simulink model "CM340A_AdcDiagc"
settings: Solver=FixedStepDiscrete  SolverMode=SingleTasking  StartTime=0.0  StopTime=1  FixedStep=0.002  RelTol=1e-3
values from neighbouring files (symbols this model uses):
  Adc0Diagc = DataDict.NTC    [CM340A_AdcDiagc_DataDict.m]
  Adc1Diagc = DataDict.NTC    [CM340A_AdcDiagc_DataDict.m]
  ADCDIAG0REFVOLT_VOLT_F32 = DataDict.Constant    [CM340A_AdcDiagc_DataDict.m]
  ADCDIAG2REFVOLT_VOLT_F32 = DataDict.Constant    [CM340A_AdcDiagc_DataDict.m]
  ADCDIAG4REFVOLT_VOLT_F32 = DataDict.Constant    [CM340A_AdcDiagc_DataDict.m]
  AdcDiagcNtc0x032FailStep = DataDict.Calibration    [CM340A_AdcDiagc_DataDict.m]
  AdcDiagcNtc0x032PassStep = DataDict.Calibration    [CM340A_AdcDiagc_DataDict.m]
  AdcDiagcNtc0x033FailStep = DataDict.Calibration    [CM340A_AdcDiagc_DataDict.m]
  AdcDiagcNtc0x033PassStep = DataDict.Calibration    [CM340A_AdcDiagc_DataDict.m]
  AdcDiagcSt = DataDict.PIM    [CM340A_AdcDiagc_DataDict.m]
  ADCDIAGPARFLTPRM_CNT_U08 = DataDict.Constant    [CM340A_AdcDiagc_DataDict.m]
  ADCDIAGSCANGROUP2REFFLTPRM_CNT_U08 = DataDict.Constant    [CM340A_AdcDiagc_DataDict.m]
  ADCDIAGSCANGROUP3REFFLTPRM_CNT_U08 = DataDict.Constant    [CM340A_AdcDiagc_DataDict.m]
  ADCDIAGSCANGROUPENDREFVOLT_VOLT_F32 = DataDict.Constant    [CM340A_AdcDiagc_DataDict.m]
  ADCDIAGSCANGROUPSTRTREFVOLT_VOLT_F32 = DataDict.Constant    [CM340A_AdcDiagc_DataDict.m]
  ADCDNECRPARERRCLR_CNT_U08 = DataDict.Constant    [CM340A_AdcDiagc_DataDict.m]
  ADCDNPERPARERRMASK_CNT_U08 = DataDict.Constant    [CM340A_AdcDiagc_DataDict.m]
  VIRTCH21_CNT_U08 = DataDict.Constant    [CM340A_AdcDiagc_DataDict.m]
  VIRTCH22_CNT_U08 = DataDict.Constant    [CM340A_AdcDiagc_DataDict.m]
  VIRTCH23_CNT_U08 = DataDict.Constant    [CM340A_AdcDiagc_DataDict.m]
undefined symbols (not defined in the file or in its folder): NtcSts1, sigbuilder_block, SigQlfr1
libraries: simulink x42, CM340A_AdcDiagc_Library x40
(part 3 of 4)

== system CM340A_AdcDiagc/AdcDiagc/AdcDiagcPer1/Adc Daigc Pointer/Strt & End Ptr Store/State 4 ==
  Action Port : ActionPort  ActionType=elseif
  Constant3 : Constant  Value=VIRTCH22_CNT_U08
  Constant4 : Constant  Value=VIRTCH22_CNT_U08
  CopyRight2 : Subsystem  Description=|  mask(Copyright Information){none=on}
      | Copyright info block.                                               
      |                                                                     
      | Place copyright information at the top of every subsystem in design.
      mask prompts: none "No parameters"
      mask help: Place copyright information at the top of every subsystem in design.
      mask Display:
      | NxtrConf = 'Nexteer Confidential';
      | 
      | sys = bdroot; %handle for the current model ("system")
      | first = get_param(sys,'Created');
      | first = first(end-3:end);  %year is last four digits
      | 
      | last = get_param(sys,'LastModifiedDate');
      | if isempty(last)
      |     last = datestr(now,'yyyy');
      | else
      |     last = last(end-3:end);
      | end
      | 
      | if strcmp(first,last)
      |     fprintf('%s -- Copyright %s Nexteer',NxtrConf,first)
      | else
      |     fprintf('%s -- %s%s- %s Nexteer',NxtrConf,char(169),first,last)
      | end
  AdcDiagcStrtPtr : Outport
  AdcDiagcEndPtr : Outport  Port=2
  wires:
  Constant3/1 -> AdcDiagcStrtPtr/1
  Constant4/1 -> AdcDiagcEndPtr/1

== system CM340A_AdcDiagc/AdcDiagc/AdcDiagcPer1/Adc Daigc Pointer/Strt & End Ptr Store/State 6 ==
  Action Port : ActionPort  ActionType=elseif
  Constant3 : Constant  Value=VIRTCH21_CNT_U08
  Constant4 : Constant  Value=VIRTCH23_CNT_U08
  CopyRight2 : Subsystem  Description=|  mask(Copyright Information){none=on}
      | Copyright info block.                                               
      |                                                                     
      | Place copyright information at the top of every subsystem in design.
      mask prompts: none "No parameters"
      mask help: Place copyright information at the top of every subsystem in design.
      mask Display:
      | NxtrConf = 'Nexteer Confidential';
      | 
      | sys = bdroot; %handle for the current model ("system")
      | first = get_param(sys,'Created');
      | first = first(end-3:end);  %year is last four digits
      | 
      | last = get_param(sys,'LastModifiedDate');
      | if isempty(last)
      |     last = datestr(now,'yyyy');
      | else
      |     last = last(end-3:end);
      | end
      | 
      | if strcmp(first,last)
      |     fprintf('%s -- Copyright %s Nexteer',NxtrConf,first)
      | else
      |     fprintf('%s -- %s%s- %s Nexteer',NxtrConf,char(169),first,last)
      | end
  AdcDiagcStrtPtr : Outport
  AdcDiagcEndPtr : Outport  Port=2
  wires:
  Constant3/1 -> AdcDiagcStrtPtr/1
  Constant4/1 -> AdcDiagcEndPtr/1

== system CM340A_AdcDiagc/AdcDiagc/AdcDiagcPer1/Adc0 Diagc/Adc0 Scan Group Strt and End Ref Voltage Diagc/CopyRight2 ==

== system CM340A_AdcDiagc/AdcDiagc/AdcDiagcPer1/Adc0 Diagc/Adc0 Scan Group Strt and End Ref Voltage Diagc/Subsystem ==
  Parameter Byte : Inport
  FltCntrPrev : Inport  Port=2
  Add : Sum
  Bitwise Operator : simulink/Logic and Bit Operations/Bitwise Operator  logicop=AND  UseBitMask=off  NumInputPorts=2  BitMask=bin2dec('01111111')  BitMaskRealWorld=Stored Integer
  Constant : Constant  Value=0
  Constant1 : Constant  Value=127  OutDataTypeStr=uint8
  CopyRight2 : Subsystem  Description=|  mask(Copyright Information){none=on}
      | Copyright info block.                                               
      |                                                                     
      | Place copyright information at the top of every subsystem in design.
      mask prompts: none "No parameters"
      mask help: Place copyright information at the top of every subsystem in design.
      mask Display:
      | NxtrConf = 'Nexteer Confidential';
      | 
      | sys = bdroot; %handle for the current model ("system")
      | first = get_param(sys,'Created');
      | first = first(end-3:end);  %year is last four digits
      | 
      | last = get_param(sys,'LastModifiedDate');
      | if isempty(last)
      |     last = datestr(now,'yyyy');
      | else
      |     last = last(end-3:end);
      | end
      | 
      | if strcmp(first,last)
      |     fprintf('%s -- Copyright %s Nexteer',NxtrConf,first)
      | else
      |     fprintf('%s -- %s%s- %s Nexteer',NxtrConf,char(169),first,last)
      | end
  Data Type Conversion2 : DataTypeConversion  OutDataTypeStr=uint8
  Relational Operator : RelationalOperator  Operator=>  OutDataTypeStr=boolean
  Scope1 : Scope  NumInputPorts=2
      settings: ShowLegends=on  TimeRange=1000  YMin=-2~0  YMax=2~256  SaveName=ScopeData3
  FltCntr : Outport
  wires:
  Constant/1 -> Relational Operator/2
  Parameter Byte/1 -> Scope1/1, Relational Operator/1
  Relational Operator/1 -> Data Type Conversion2/1
  Add/1 -> Bitwise Operator/1
  Bitwise Operator/1 -> FltCntr/1, Scope1/2
  FltCntrPrev/1 -> Add/2
  Data Type Conversion2/1 -> Add/1
  Constant1/1 -> Bitwise Operator/2

== system CM340A_AdcDiagc/AdcDiagc/AdcDiagcPer1/Adc0 Diagc/Adc0 Scan Group Strt and End Ref Voltage Diagc/Subsystem1 ==
  Parameter Byte : Inport
  FltCntrPrev : Inport  Port=2
  Add : Sum
  Bitwise Operator : simulink/Logic and Bit Operations/Bitwise Operator  logicop=AND  UseBitMask=off  NumInputPorts=2  BitMask=bin2dec('01111111')  BitMaskRealWorld=Stored Integer
  Constant : Constant  Value=0
  Constant1 : Constant  Value=127  OutDataTypeStr=uint8
  CopyRight2 : Subsystem  Description=|  mask(Copyright Information){none=on}
      | Copyright info block.                                               
      |                                                                     
      | Place copyright information at the top of every subsystem in design.
      mask prompts: none "No parameters"
      mask help: Place copyright information at the top of every subsystem in design.
      mask Display:
      | NxtrConf = 'Nexteer Confidential';
      | 
      | sys = bdroot; %handle for the current model ("system")
      | first = get_param(sys,'Created');
      | first = first(end-3:end);  %year is last four digits
      | 
      | last = get_param(sys,'LastModifiedDate');
      | if isempty(last)
      |     last = datestr(now,'yyyy');
      | else
      |     last = last(end-3:end);
      | end
      | 
      | if strcmp(first,last)
      |     fprintf('%s -- Copyright %s Nexteer',NxtrConf,first)
      | else
      |     fprintf('%s -- %s%s- %s Nexteer',NxtrConf,char(169),first,last)
      | end
  Data Type Conversion2 : DataTypeConversion  OutDataTypeStr=uint8
  Relational Operator : RelationalOperator  Operator=>  OutDataTypeStr=boolean
  Scope1 : Scope  NumInputPorts=2
      settings: ShowLegends=on  TimeRange=1000  YMin=-2~0  YMax=2~256  SaveName=ScopeData4
  FltCntr : Outport
  wires:
  Constant/1 -> Relational Operator/2
  Parameter Byte/1 -> Scope1/1, Relational Operator/1
  Relational Operator/1 -> Data Type Conversion2/1
  Add/1 -> Bitwise Operator/1
  Bitwise Operator/1 -> FltCntr/1, Scope1/2
  FltCntrPrev/1 -> Add/2
  Data Type Conversion2/1 -> Add/1
  Constant1/1 -> Bitwise Operator/2

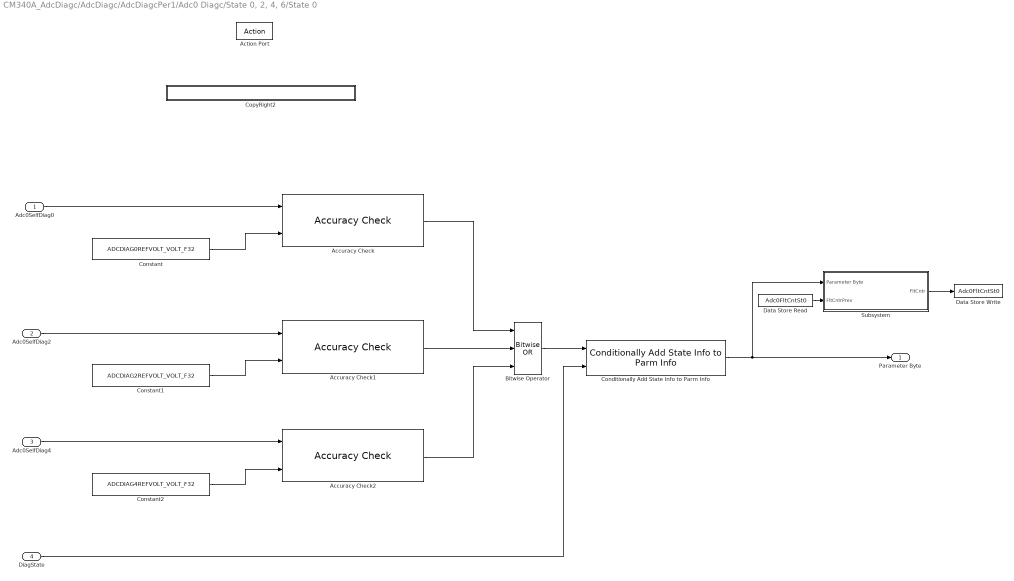
== system CM340A_AdcDiagc/AdcDiagc/AdcDiagcPer1/Adc0 Diagc/State 0, 2, 4, 6/State 0 ==
  Adc0SelfDiag0 : Inport  RequirementInfo={} %GIDa_a23626af_39b5_4ed6_8e27_9b4935a63c0c
  Adc0SelfDiag2 : Inport  RequirementInfo={} %GIDa_c5f8a541_29c5_4f9c_88e4_ee09e309bb5e  Port=2
  Adc0SelfDiag4 : Inport  RequirementInfo={} %GIDa_cb51580b_1e3d_432c_bc7e_60394d016f61  Port=3
  DiagState : Inport  Port=4
  Action Port : ActionPort  ActionType=then
  Accuracy Check : CM340A_AdcDiagc_Library/Accuracy Check  RequirementInfo="{'linktype_rmi_doors' '000079f2 (/ESG Group/FDD Module Requirements/EA4 Specific/CM340A_AdcDiagc)' '#CM340A_190' 'true' 'REQ:  CM340A_190' '' } %GIDa_1e4f0f1f_efcc_4971_978e_b5150d55866c"
  Accuracy Check1 : CM340A_AdcDiagc_Library/Accuracy Check  RequirementInfo="{'linktype_rmi_doors' '000079f2 (/ESG Group/FDD Module Requirements/EA4 Specific/CM340A_AdcDiagc)' '#CM340A_191' 'true' 'REQ:  CM340A_191' '' } %GIDa_c4102599_b47c_4dea_9090_c33325f35ddf"
  Accuracy Check2 : CM340A_AdcDiagc_Library/Accuracy Check  RequirementInfo="{'linktype_rmi_doors' '000079f2 (/ESG Group/FDD Module Requirements/EA4 Specific/CM340A_AdcDiagc)' '#CM340A_192' 'true' 'REQ:  CM340A_192' '' } %GIDa_02166258_10fd_4a19_8760_8d3e602927dd"
  Bitwise Operator : simulink/Logic and Bit Operations/Bitwise Operator  logicop=OR  UseBitMask=off  NumInputPorts=3  BitMask=bin2dec('11011001')  BitMaskRealWorld=Stored Integer
  Conditionally Add State Info to Parm Info : CM340A_AdcDiagc_Library/Conditionally Add State Info to Parm Info  RequirementInfo="{'linktype_rmi_doors' '000079f2 (/ESG Group/FDD Module Requirements/EA4 Specific/CM340A_AdcDiagc)' '#CM340A_173' 'true' 'REQ:  CM340A_173' '' } %GIDa_80ab0b66_9e6f_4bf7_ac53_ccce88f803b6"
  Constant : Constant  Value=ADCDIAG0REFVOLT_VOLT_F32
  Constant1 : Constant  Value=ADCDIAG2REFVOLT_VOLT_F32
  Constant2 : Constant  Value=ADCDIAG4REFVOLT_VOLT_F32
  CopyRight2 : Subsystem  Description=|  mask(Copyright Information){none=on}
      | Copyright info block.                                               
      |                                                                     
      | Place copyright information at the top of every subsystem in design.
      mask prompts: none "No parameters"
      mask help: Place copyright information at the top of every subsystem in design.
      mask Display:
      | NxtrConf = 'Nexteer Confidential';
      | 
      | sys = bdroot; %handle for the current model ("system")
      | first = get_param(sys,'Created');
      | first = first(end-3:end);  %year is last four digits
      | 
      | last = get_param(sys,'LastModifiedDate');
      | if isempty(last)
      |     last = datestr(now,'yyyy');
      | else
      |     last = last(end-3:end);
      | end
      | 
      | if strcmp(first,last)
      |     fprintf('%s -- Copyright %s Nexteer',NxtrConf,first)
      | else
      |     fprintf('%s -- %s%s- %s Nexteer',NxtrConf,char(169),first,last)
      | end
  Data Store Read : DataStoreRead  DataStoreName=Adc0FltCntSt0
  Data Store Write : DataStoreWrite  DataStoreName=Adc0FltCntSt0
  Subsystem : Subsystem
  Parameter Byte : Outport
  wires:
  Adc0SelfDiag0/1 -> Accuracy Check/1
  Constant/1 -> Accuracy Check/2
  Adc0SelfDiag2/1 -> Accuracy Check1/1
  Constant1/1 -> Accuracy Check1/2
  Adc0SelfDiag4/1 -> Accuracy Check2/1
  Constant2/1 -> Accuracy Check2/2
  Accuracy Check/1 -> Bitwise Operator/1
  Accuracy Check1/1 -> Bitwise Operator/2
  Accuracy Check2/1 -> Bitwise Operator/3
  Conditionally Add State Info to Parm Info/1 -> Subsystem/1(Parameter Byte), Parameter Byte/1
  Subsystem/1(FltCntr) -> Data Store Write/1
  Data Store Read/1 -> Subsystem/2(FltCntrPrev)
  DiagState/1 -> Conditionally Add State Info to Parm Info/2
  Bitwise Operator/1 -> Conditionally Add State Info to Parm Info/1

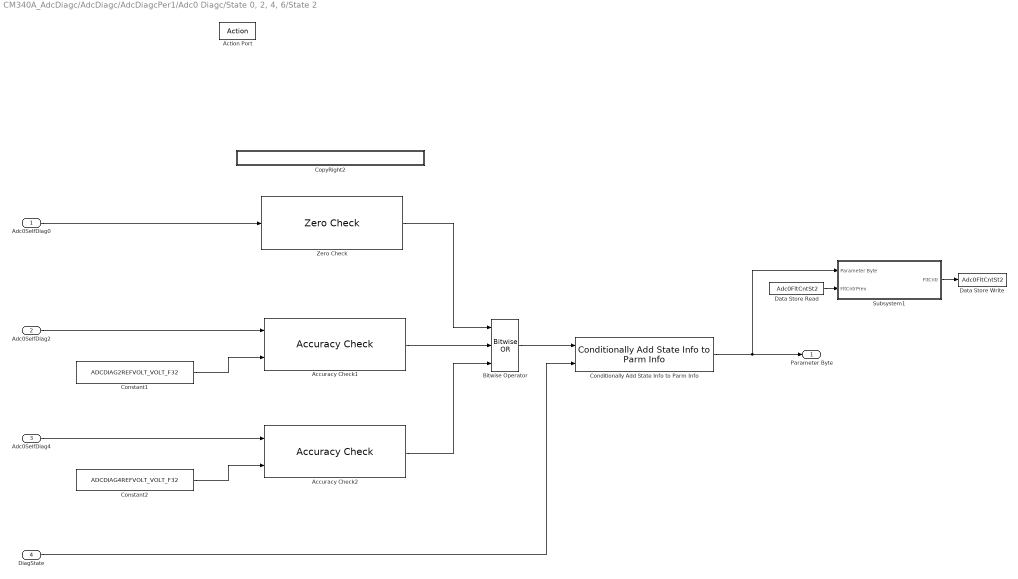
== system CM340A_AdcDiagc/AdcDiagc/AdcDiagcPer1/Adc0 Diagc/State 0, 2, 4, 6/State 2 ==
  Adc0SelfDiag0 : Inport  RequirementInfo={} %GIDa_e1135336_cc92_42c6_b177_9493a56e2976
  Adc0SelfDiag2 : Inport  RequirementInfo={} %GIDa_5cb7465b_8501_4efa_b631_17bf9f2d25f9  Port=2
  Adc0SelfDiag4 : Inport  RequirementInfo={} %GIDa_b0fa7dd1_c197_4d64_b6d1_f806bb0091d3  Port=3
  DiagState : Inport  Port=4
  Action Port : ActionPort  ActionType=elseif
  Accuracy Check1 : CM340A_AdcDiagc_Library/Accuracy Check  RequirementInfo="{'linktype_rmi_doors' '000079f2 (/ESG Group/FDD Module Requirements/EA4 Specific/CM340A_AdcDiagc)' '#CM340A_98' 'true' 'REQ:  CM340A_98' '' } %GIDa_e4dc49a1_cd8d_4004_aa7e_ba9570b56871"
  Accuracy Check2 : CM340A_AdcDiagc_Library/Accuracy Check  RequirementInfo="{'linktype_rmi_doors' '000079f2 (/ESG Group/FDD Module Requirements/EA4 Specific/CM340A_AdcDiagc)' '#CM340A_99' 'true' 'REQ:  CM340A_99' '' } %GIDa_6f3293bb_0d9c_4093_8771_c0457607681b"
  Bitwise Operator : simulink/Logic and Bit Operations/Bitwise Operator  logicop=OR  UseBitMask=off  NumInputPorts=3  BitMask=bin2dec('11011001')  BitMaskRealWorld=Stored Integer
  Conditionally Add State Info to Parm Info : CM340A_AdcDiagc_Library/Conditionally Add State Info to Parm Info  RequirementInfo="{'linktype_rmi_doors' '000079f2 (/ESG Group/FDD Module Requirements/EA4 Specific/CM340A_AdcDiagc)' '#CM340A_173' 'true' 'REQ:  CM340A_173' '' } %GIDa_c444345b_0a68_47e3_89f4_ca02f2b76309"
  Constant1 : Constant  Value=ADCDIAG2REFVOLT_VOLT_F32
  Constant2 : Constant  Value=ADCDIAG4REFVOLT_VOLT_F32
  CopyRight2 : Subsystem  Description=|  mask(Copyright Information){none=on}
      | Copyright info block.                                               
      |                                                                     
      | Place copyright information at the top of every subsystem in design.
      mask prompts: none "No parameters"
      mask help: Place copyright information at the top of every subsystem in design.
      mask Display:
      | NxtrConf = 'Nexteer Confidential';
      | 
      | sys = bdroot; %handle for the current model ("system")
      | first = get_param(sys,'Created');
      | first = first(end-3:end);  %year is last four digits
      | 
      | last = get_param(sys,'LastModifiedDate');
      | if isempty(last)
      |     last = datestr(now,'yyyy');
      | else
      |     last = last(end-3:end);
      | end
      | 
      | if strcmp(first,last)
      |     fprintf('%s -- Copyright %s Nexteer',NxtrConf,first)
      | else
      |     fprintf('%s -- %s%s- %s Nexteer',NxtrConf,char(169),first,last)
      | end
  Data Store Read : DataStoreRead  DataStoreName=Adc0FltCntSt2
  Data Store Write : DataStoreWrite  DataStoreName=Adc0FltCntSt2
  Subsystem1 : Subsystem
  Zero Check : CM340A_AdcDiagc_Library/Zero Check  RequirementInfo="{'linktype_rmi_doors' '000079f2 (/ESG Group/FDD Module Requirements/EA4 Specific/CM340A_AdcDiagc)' '#CM340A_97' 'true' 'REQ:  CM340A_97' '' } %GIDa_0e901c83_9a28_413b_b5d3_3d84a5c12599"
  Parameter Byte : Outport
  wires:
  Accuracy Check2/1 -> Bitwise Operator/3
  Accuracy Check1/1 -> Bitwise Operator/2
  Zero Check/1 -> Bitwise Operator/1
  Constant2/1 -> Accuracy Check2/2
  Adc0SelfDiag4/1 -> Accuracy Check2/1
  Constant1/1 -> Accuracy Check1/2
  Adc0SelfDiag2/1 -> Accuracy Check1/1
  Adc0SelfDiag0/1 -> Zero Check/1
  Conditionally Add State Info to Parm Info/1 -> Subsystem1/1(Parameter Byte), Parameter Byte/1
  Subsystem1/1(FltCntr) -> Data Store Write/1
  Data Store Read/1 -> Subsystem1/2(FltCntrPrev)
  DiagState/1 -> Conditionally Add State Info to Parm Info/2
  Bitwise Operator/1 -> Conditionally Add State Info to Parm Info/1

== system CM340A_AdcDiagc/AdcDiagc/AdcDiagcPer1/Adc0 Diagc/State 0, 2, 4, 6/State 4 ==
  Adc0SelfDiag0 : Inport  RequirementInfo={} %GIDa_80669d4d_c17e_4351_968c_a5cdc73e2fd0
  Adc0SelfDiag2 : Inport  RequirementInfo={} %GIDa_5478fd37_db90_473f_8f3a_3f32002dca06  Port=2
  Adc0SelfDiag4 : Inport  RequirementInfo={} %GIDa_29685fa4_30be_4985_ab67_87372302ea4d  Port=3
  DiagState : Inport  Port=4
  Action Port : ActionPort  ActionType=elseif
  Accuracy Check2 : CM340A_AdcDiagc_Library/Accuracy Check  RequirementInfo="{'linktype_rmi_doors' '000079f2 (/ESG Group/FDD Module Requirements/EA4 Specific/CM340A_AdcDiagc)' '#CM340A_109' 'true' 'REQ:  CM340A_109' '' } %GIDa_6c183749_093e_44f2_b8e4_facecc57cf84"
  Bitwise Operator : simulink/Logic and Bit Operations/Bitwise Operator  logicop=OR  UseBitMask=off  NumInputPorts=3  BitMask=bin2dec('11011001')  BitMaskRealWorld=Stored Integer
  Conditionally Add State Info to Parm Info : CM340A_AdcDiagc_Library/Conditionally Add State Info to Parm Info  RequirementInfo="{'linktype_rmi_doors' '000079f2 (/ESG Group/FDD Module Requirements/EA4 Specific/CM340A_AdcDiagc)' '#CM340A_173' 'true' 'REQ:  CM340A_173' '' } %GIDa_b77621d8_fa12_4826_8388_96ac13845245"
  Constant2 : Constant  Value=ADCDIAG4REFVOLT_VOLT_F32
  CopyRight2 : Subsystem  Description=|  mask(Copyright Information){none=on}
      | Copyright info block.                                               
      |                                                                     
      | Place copyright information at the top of every subsystem in design.
      mask prompts: none "No parameters"
      mask help: Place copyright information at the top of every subsystem in design.
      mask Display:
      | NxtrConf = 'Nexteer Confidential';
      | 
      | sys = bdroot; %handle for the current model ("system")
      | first = get_param(sys,'Created');
      | first = first(end-3:end);  %year is last four digits
      | 
      | last = get_param(sys,'LastModifiedDate');
      | if isempty(last)
      |     last = datestr(now,'yyyy');
      | else
      |     last = last(end-3:end);
      | end
      | 
      | if strcmp(first,last)
      |     fprintf('%s -- Copyright %s Nexteer',NxtrConf,first)
      | else
      |     fprintf('%s -- %s%s- %s Nexteer',NxtrConf,char(169),first,last)
      | end
  Data Store Read : DataStoreRead  DataStoreName=Adc0FltCntSt4
  Data Store Write : DataStoreWrite  DataStoreName=Adc0FltCntSt4
  Subsystem : Subsystem
  Zero Check : CM340A_AdcDiagc_Library/Zero Check  RequirementInfo="{'linktype_rmi_doors' '000079f2 (/ESG Group/FDD Module Requirements/EA4 Specific/CM340A_AdcDiagc)' '#CM340A_107' 'true' 'REQ:  CM340A_107' '' } %GIDa_5caf8c48_9578_4a46_a60d_91b9ca66570e"
  Zero Check1 : CM340A_AdcDiagc_Library/Zero Check  RequirementInfo="{'linktype_rmi_doors' '000079f2 (/ESG Group/FDD Module Requirements/EA4 Specific/CM340A_AdcDiagc)' '#CM340A_108' 'true' 'REQ:  CM340A_108' '' } %GIDa_44885def_83bb_498b_a6ad_cca791d96317"
  Parameter Byte : Outport
  wires:
  Accuracy Check2/1 -> Bitwise Operator/3
  Zero Check1/1 -> Bitwise Operator/2
  Zero Check/1 -> Bitwise Operator/1
  Constant2/1 -> Accuracy Check2/2
  Adc0SelfDiag4/1 -> Accuracy Check2/1
  Adc0SelfDiag2/1 -> Zero Check1/1
  Adc0SelfDiag0/1 -> Zero Check/1
  Conditionally Add State Info to Parm Info/1 -> Subsystem/1(Parameter Byte), Parameter Byte/1
  Subsystem/1(FltCntr) -> Data Store Write/1
  Data Store Read/1 -> Subsystem/2(FltCntrPrev)
  DiagState/1 -> Conditionally Add State Info to Parm Info/2
  Bitwise Operator/1 -> Conditionally Add State Info to Parm Info/1

== system CM340A_AdcDiagc/AdcDiagc/AdcDiagcPer1/Adc0 Diagc/State 0, 2, 4, 6/State 6 ==
  Adc0SelfDiag0 : Inport  RequirementInfo={} %GIDa_cc6bfecf_eb36_4463_85fc_a6e32f107854
  Adc0SelfDiag2 : Inport  RequirementInfo={} %GIDa_b01f49d9_401a_4125_b929_3202f5b0e65e  Port=2
  Adc0SelfDiag4 : Inport  RequirementInfo={} %GIDa_56e02736_13f5_48bd_b42c_fe10036a1660  Port=3
  DiagState : Inport  Port=4
  Action Port : ActionPort  ActionType=else
  Accuracy Check1 : CM340A_AdcDiagc_Library/Accuracy Check  RequirementInfo="{'linktype_rmi_doors' '000079f2 (/ESG Group/FDD Module Requirements/EA4 Specific/CM340A_AdcDiagc)' '#CM340A_117' 'true' 'REQ:  CM340A_117' '' } %GIDa_9d9fd4e8_190d_495f_8add_1c2530f0c5ec"
  Bitwise Operator : simulink/Logic and Bit Operations/Bitwise Operator  logicop=OR  UseBitMask=off  NumInputPorts=3  BitMask=bin2dec('11011001')  BitMaskRealWorld=Stored Integer
  Conditionally Add State Info to Parm Info : CM340A_AdcDiagc_Library/Conditionally Add State Info to Parm Info  RequirementInfo="{'linktype_rmi_doors' '000079f2 (/ESG Group/FDD Module Requirements/EA4 Specific/CM340A_AdcDiagc)' '#CM340A_173' 'true' 'REQ:  CM340A_173' '' } %GIDa_f744b400_d67c_429e_a861_24a05740f070"
  Constant1 : Constant  Value=ADCDIAG2REFVOLT_VOLT_F32
  CopyRight2 : Subsystem  Description=|  mask(Copyright Information){none=on}
      | Copyright info block.                                               
      |                                                                     
      | Place copyright information at the top of every subsystem in design.
      mask prompts: none "No parameters"
      mask help: Place copyright information at the top of every subsystem in design.
      mask Display:
      | NxtrConf = 'Nexteer Confidential';
      | 
      | sys = bdroot; %handle for the current model ("system")
      | first = get_param(sys,'Created');
      | first = first(end-3:end);  %year is last four digits
      | 
      | last = get_param(sys,'LastModifiedDate');
      | if isempty(last)
      |     last = datestr(now,'yyyy');
      | else
      |     last = last(end-3:end);
      | end
      | 
      | if strcmp(first,last)
      |     fprintf('%s -- Copyright %s Nexteer',NxtrConf,first)
      | else
      |     fprintf('%s -- %s%s- %s Nexteer',NxtrConf,char(169),first,last)
      | end
  Data Store Read : DataStoreRead  DataStoreName=Adc0FltCntSt6
  Data Store Write : DataStoreWrite  DataStoreName=Adc0FltCntSt6
  Subsystem : Subsystem
  Zero Check : CM340A_AdcDiagc_Library/Zero Check  RequirementInfo="{'linktype_rmi_doors' '000079f2 (/ESG Group/FDD Module Requirements/EA4 Specific/CM340A_AdcDiagc)' '#CM340A_116' 'true' 'REQ:  CM340A_116' '' } %GIDa_f3ee25d7_da18_40a6_80b3_4e69cb85b376"
  Zero Check1 : CM340A_AdcDiagc_Library/Zero Check  RequirementInfo="{'linktype_rmi_doors' '000079f2 (/ESG Group/FDD Module Requirements/EA4 Specific/CM340A_AdcDiagc)' '#CM340A_118' 'true' 'REQ:  CM340A_118' '' } %GIDa_612deb41_1d94_4982_964c_6f195a5afc4b"
  Parameter Byte : Outport
  wires:
  Adc0SelfDiag0/1 -> Zero Check/1
  Adc0SelfDiag2/1 -> Accuracy Check1/1
  Constant1/1 -> Accuracy Check1/2
  Adc0SelfDiag4/1 -> Zero Check1/1
  Zero Check/1 -> Bitwise Operator/1
  Accuracy Check1/1 -> Bitwise Operator/2
  Zero Check1/1 -> Bitwise Operator/3
  Conditionally Add State Info to Parm Info/1 -> Subsystem/1(Parameter Byte), Parameter Byte/1
  Subsystem/1(FltCntr) -> Data Store Write/1
  Data Store Read/1 -> Subsystem/2(FltCntrPrev)
  DiagState/1 -> Conditionally Add State Info to Parm Info/2
  Bitwise Operator/1 -> Conditionally Add State Info to Parm Info/1

== system CM340A_AdcDiagc/AdcDiagc/AdcDiagcPer1/Adc0 Diagc/State 1,3,5,7/CopyRight2 ==

== system CM340A_AdcDiagc/AdcDiagc/AdcDiagcPer1/Adc1 Diagc/Adc1 Scan Group Strt and End Ref Voltage Diagc/CopyRight2 ==

== system CM340A_AdcDiagc/AdcDiagc/AdcDiagcPer1/Adc1 Diagc/Adc1 Scan Group Strt and End Ref Voltage Diagc/Subsystem ==
  Parameter Byte : Inport
  FltCntrPrev : Inport  Port=2
  Add : Sum
  Bitwise Operator : simulink/Logic and Bit Operations/Bitwise Operator  logicop=AND  UseBitMask=off  NumInputPorts=2  BitMask=bin2dec('01111111')  BitMaskRealWorld=Stored Integer
  Constant : Constant  Value=0
  Constant1 : Constant  Value=127  OutDataTypeStr=uint8
  CopyRight2 : Subsystem  Description=|  mask(Copyright Information){none=on}
      | Copyright info block.                                               
      |                                                                     
      | Place copyright information at the top of every subsystem in design.
      mask prompts: none "No parameters"
      mask help: Place copyright information at the top of every subsystem in design.
      mask Display:
      | NxtrConf = 'Nexteer Confidential';
      | 
      | sys = bdroot; %handle for the current model ("system")
      | first = get_param(sys,'Created');
      | first = first(end-3:end);  %year is last four digits
      | 
      | last = get_param(sys,'LastModifiedDate');
      | if isempty(last)
      |     last = datestr(now,'yyyy');
      | else
      |     last = last(end-3:end);
      | end
      | 
      | if strcmp(first,last)
      |     fprintf('%s -- Copyright %s Nexteer',NxtrConf,first)
      | else
      |     fprintf('%s -- %s%s- %s Nexteer',NxtrConf,char(169),first,last)
      | end
  Data Type Conversion2 : DataTypeConversion  OutDataTypeStr=uint8
  Relational Operator : RelationalOperator  Operator=>  OutDataTypeStr=boolean
  Scope1 : Scope  NumInputPorts=2
      settings: ShowLegends=on  TimeRange=1000  YMin=-2~0  YMax=2~256  SaveName=ScopeData6
  FltCntr : Outport
  wires:
  Constant/1 -> Relational Operator/2
  Parameter Byte/1 -> Scope1/1, Relational Operator/1
  Relational Operator/1 -> Data Type Conversion2/1
  Add/1 -> Bitwise Operator/1
  Bitwise Operator/1 -> FltCntr/1, Scope1/2
  FltCntrPrev/1 -> Add/2
  Data Type Conversion2/1 -> Add/1
  Constant1/1 -> Bitwise Operator/2

== system CM340A_AdcDiagc/AdcDiagc/AdcDiagcPer1/Adc1 Diagc/Adc1 Scan Group Strt and End Ref Voltage Diagc/Subsystem1 ==
  Parameter Byte : Inport
  FltCntrPrev : Inport  Port=2
  Add : Sum
  Bitwise Operator : simulink/Logic and Bit Operations/Bitwise Operator  logicop=AND  UseBitMask=off  NumInputPorts=2  BitMask=bin2dec('01111111')  BitMaskRealWorld=Stored Integer
  Constant : Constant  Value=0
  Constant1 : Constant  Value=127  OutDataTypeStr=uint8
  CopyRight2 : Subsystem  Description=|  mask(Copyright Information){none=on}
      | Copyright info block.                                               
      |                                                                     
      | Place copyright information at the top of every subsystem in design.
      mask prompts: none "No parameters"
      mask help: Place copyright information at the top of every subsystem in design.
      mask Display:
      | NxtrConf = 'Nexteer Confidential';
      | 
      | sys = bdroot; %handle for the current model ("system")
      | first = get_param(sys,'Created');
      | first = first(end-3:end);  %year is last four digits
      | 
      | last = get_param(sys,'LastModifiedDate');
      | if isempty(last)
      |     last = datestr(now,'yyyy');
      | else
      |     last = last(end-3:end);
      | end
      | 
      | if strcmp(first,last)
      |     fprintf('%s -- Copyright %s Nexteer',NxtrConf,first)
      | else
      |     fprintf('%s -- %s%s- %s Nexteer',NxtrConf,char(169),first,last)
      | end
  Data Type Conversion2 : DataTypeConversion  OutDataTypeStr=uint8
  Relational Operator : RelationalOperator  Operator=>  OutDataTypeStr=boolean
  Scope1 : Scope  NumInputPorts=2
      settings: ShowLegends=on  TimeRange=1000  YMin=-2~0  YMax=2~256  SaveName=ScopeData7
  FltCntr : Outport
  wires:
  Constant/1 -> Relational Operator/2
  Parameter Byte/1 -> Scope1/1, Relational Operator/1
  Relational Operator/1 -> Data Type Conversion2/1
  Add/1 -> Bitwise Operator/1
  Bitwise Operator/1 -> FltCntr/1, Scope1/2
  FltCntrPrev/1 -> Add/2
  Data Type Conversion2/1 -> Add/1
  Constant1/1 -> Bitwise Operator/2

== system CM340A_AdcDiagc/AdcDiagc/AdcDiagcPer1/Adc1 Diagc/State 0,2,4,6/CopyRight2 ==

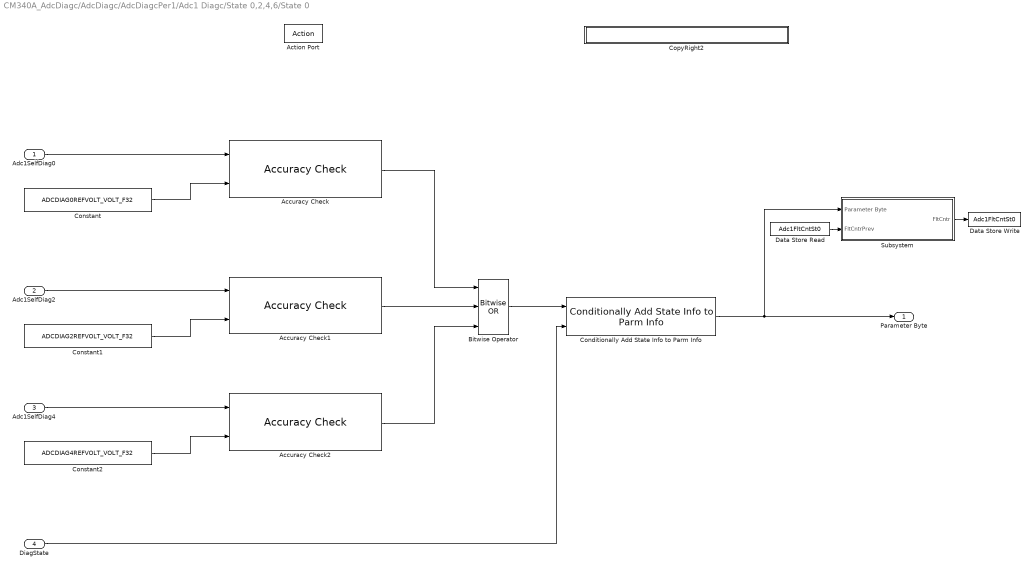
== system CM340A_AdcDiagc/AdcDiagc/AdcDiagcPer1/Adc1 Diagc/State 0,2,4,6/State 0 ==
  Adc1SelfDiag0 : Inport  RequirementInfo={} %GIDa_5e96d837_e748_4f74_be6c_ec57e578337d
  Adc1SelfDiag2 : Inport  RequirementInfo={} %GIDa_5d9abc12_bee9_4b89_83e8_316962194616  Port=2
  Adc1SelfDiag4 : Inport  RequirementInfo={} %GIDa_c6d973ad_72cd_4735_bb5d_43ae1fb43be0  Port=3
  DiagState : Inport  Port=4
  Action Port : ActionPort  ActionType=then
  Accuracy Check : CM340A_AdcDiagc_Library/Accuracy Check  RequirementInfo="{'linktype_rmi_doors' '000079f2 (/ESG Group/FDD Module Requirements/EA4 Specific/CM340A_AdcDiagc)' '#CM340A_144' 'true' 'REQ:  CM340A_144' '' } %GIDa_38e85564_4b0e_4e45_ab03_60e54ef8070c"
  Accuracy Check1 : CM340A_AdcDiagc_Library/Accuracy Check  RequirementInfo="{'linktype_rmi_doors' '000079f2 (/ESG Group/FDD Module Requirements/EA4 Specific/CM340A_AdcDiagc)' '#CM340A_145' 'true' 'REQ:  CM340A_145' '' } %GIDa_abe12da3_1bd6_49b0_ab3e_a63855ab3f6f"
  Accuracy Check2 : CM340A_AdcDiagc_Library/Accuracy Check  RequirementInfo="{'linktype_rmi_doors' '000079f2 (/ESG Group/FDD Module Requirements/EA4 Specific/CM340A_AdcDiagc)' '#CM340A_146' 'true' 'REQ:  CM340A_146' '' } %GIDa_bb769c91_cbb0_4b85_b90b_6235162b78b0"
  Bitwise Operator : simulink/Logic and Bit Operations/Bitwise Operator  logicop=OR  UseBitMask=off  NumInputPorts=3  BitMask=bin2dec('11011001')  BitMaskRealWorld=Stored Integer
  Conditionally Add State Info to Parm Info : CM340A_AdcDiagc_Library/Conditionally Add State Info to Parm Info  RequirementInfo="{'linktype_rmi_doors' '000079f2 (/ESG Group/FDD Module Requirements/EA4 Specific/CM340A_AdcDiagc)' '#CM340A_173' 'true' 'REQ:  CM340A_173' '' } %GIDa_48bc11a5_b758_450f_a5d6_f0cdd3b6ec5f"
  Constant : Constant  Value=ADCDIAG0REFVOLT_VOLT_F32
  Constant1 : Constant  Value=ADCDIAG2REFVOLT_VOLT_F32
  Constant2 : Constant  Value=ADCDIAG4REFVOLT_VOLT_F32
  CopyRight2 : Subsystem  Description=|  mask(Copyright Information){none=on}
      | Copyright info block.                                               
      |                                                                     
      | Place copyright information at the top of every subsystem in design.
      mask prompts: none "No parameters"
      mask help: Place copyright information at the top of every subsystem in design.
      mask Display:
      | NxtrConf = 'Nexteer Confidential';
      | 
      | sys = bdroot; %handle for the current model ("system")
      | first = get_param(sys,'Created');
      | first = first(end-3:end);  %year is last four digits
      | 
      | last = get_param(sys,'LastModifiedDate');
      | if isempty(last)
      |     last = datestr(now,'yyyy');
      | else
      |     last = last(end-3:end);
      | end
      | 
      | if strcmp(first,last)
      |     fprintf('%s -- Copyright %s Nexteer',NxtrConf,first)
      | else
      |     fprintf('%s -- %s%s- %s Nexteer',NxtrConf,char(169),first,last)
      | end
  Data Store Read : DataStoreRead  DataStoreName=Adc1FltCntSt0
  Data Store Write : DataStoreWrite  DataStoreName=Adc1FltCntSt0
  Subsystem : Subsystem
  Parameter Byte : Outport
  wires:
  Accuracy Check2/1 -> Bitwise Operator/3
  Accuracy Check1/1 -> Bitwise Operator/2
  Accuracy Check/1 -> Bitwise Operator/1
  Constant2/1 -> Accuracy Check2/2
  Adc1SelfDiag4/1 -> Accuracy Check2/1
  Constant1/1 -> Accuracy Check1/2
  Adc1SelfDiag2/1 -> Accuracy Check1/1
  Constant/1 -> Accuracy Check/2
  Adc1SelfDiag0/1 -> Accuracy Check/1
  Conditionally Add State Info to Parm Info/1 -> Subsystem/1(Parameter Byte), Parameter Byte/1
  Subsystem/1(FltCntr) -> Data Store Write/1
  Data Store Read/1 -> Subsystem/2(FltCntrPrev)
  DiagState/1 -> Conditionally Add State Info to Parm Info/2
  Bitwise Operator/1 -> Conditionally Add State Info to Parm Info/1

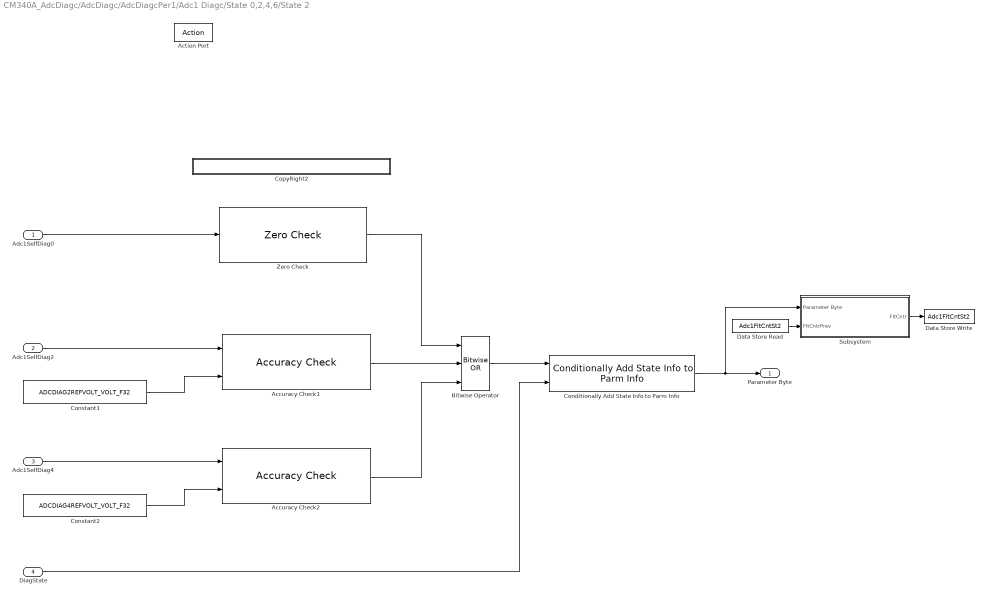
== system CM340A_AdcDiagc/AdcDiagc/AdcDiagcPer1/Adc1 Diagc/State 0,2,4,6/State 2 ==
  Adc1SelfDiag0 : Inport  RequirementInfo={} %GIDa_b183a0d3_d87b_4723_8df9_4d0ccb6c8bee
  Adc1SelfDiag2 : Inport  RequirementInfo={} %GIDa_535d0c0b_2ec1_4e0d_96ee_68160d37cae3  Port=2
  Adc1SelfDiag4 : Inport  RequirementInfo={} %GIDa_dd172795_af9b_4600_9299_e051c4385c50  Port=3
  DiagState : Inport  Port=4
  Action Port : ActionPort  ActionType=elseif
  Accuracy Check1 : CM340A_AdcDiagc_Library/Accuracy Check  RequirementInfo="{'linktype_rmi_doors' '000079f2 (/ESG Group/FDD Module Requirements/EA4 Specific/CM340A_AdcDiagc)' '#CM340A_153' 'true' 'REQ:  CM340A_153' '' } %GIDa_6a88b810_477b_4def_963b_4fea408449f6"
  Accuracy Check2 : CM340A_AdcDiagc_Library/Accuracy Check  RequirementInfo="{'linktype_rmi_doors' '000079f2 (/ESG Group/FDD Module Requirements/EA4 Specific/CM340A_AdcDiagc)' '#CM340A_154' 'true' 'REQ:  CM340A_154' '' } %GIDa_9bc39c3c_cd17_48da_8192_772b3df82507"
  Bitwise Operator : simulink/Logic and Bit Operations/Bitwise Operator  logicop=OR  UseBitMask=off  NumInputPorts=3  BitMask=bin2dec('11011001')  BitMaskRealWorld=Stored Integer
  Conditionally Add State Info to Parm Info : CM340A_AdcDiagc_Library/Conditionally Add State Info to Parm Info  RequirementInfo="{'linktype_rmi_doors' '000079f2 (/ESG Group/FDD Module Requirements/EA4 Specific/CM340A_AdcDiagc)' '#CM340A_173' 'true' 'REQ:  CM340A_173' '' } %GIDa_6561668f_3868_4276_a6a7_fefe2d045dc5"
  Constant1 : Constant  Value=ADCDIAG2REFVOLT_VOLT_F32
  Constant2 : Constant  Value=ADCDIAG4REFVOLT_VOLT_F32
  CopyRight2 : Subsystem  Description=|  mask(Copyright Information){none=on}
      | Copyright info block.                                               
      |                                                                     
      | Place copyright information at the top of every subsystem in design.
      mask prompts: none "No parameters"
      mask help: Place copyright information at the top of every subsystem in design.
      mask Display:
      | NxtrConf = 'Nexteer Confidential';
      | 
      | sys = bdroot; %handle for the current model ("system")
      | first = get_param(sys,'Created');
      | first = first(end-3:end);  %year is last four digits
      | 
      | last = get_param(sys,'LastModifiedDate');
      | if isempty(last)
      |     last = datestr(now,'yyyy');
      | else
      |     last = last(end-3:end);
      | end
      | 
      | if strcmp(first,last)
      |     fprintf('%s -- Copyright %s Nexteer',NxtrConf,first)
      | else
      |     fprintf('%s -- %s%s- %s Nexteer',NxtrConf,char(169),first,last)
      | end
  Data Store Read : DataStoreRead  DataStoreName=Adc1FltCntSt2
  Data Store Write : DataStoreWrite  DataStoreName=Adc1FltCntSt2
  Subsystem : Subsystem
  Zero Check : CM340A_AdcDiagc_Library/Zero Check  RequirementInfo="{'linktype_rmi_doors' '000079f2 (/ESG Group/FDD Module Requirements/EA4 Specific/CM340A_AdcDiagc)' '#CM340A_152' 'true' 'REQ:  CM340A_152' '' } %GIDa_d0df1a3e_6067_468e_877f_2eda52c61916"
  Parameter Byte : Outport
  wires:
  Adc1SelfDiag0/1 -> Zero Check/1
  Adc1SelfDiag2/1 -> Accuracy Check1/1
  Constant1/1 -> Accuracy Check1/2
  Adc1SelfDiag4/1 -> Accuracy Check2/1
  Constant2/1 -> Accuracy Check2/2
  Zero Check/1 -> Bitwise Operator/1
  Accuracy Check1/1 -> Bitwise Operator/2
  Accuracy Check2/1 -> Bitwise Operator/3
  Conditionally Add State Info to Parm Info/1 -> Subsystem/1(Parameter Byte), Parameter Byte/1
  Subsystem/1(FltCntr) -> Data Store Write/1
  Data Store Read/1 -> Subsystem/2(FltCntrPrev)
  DiagState/1 -> Conditionally Add State Info to Parm Info/2
  Bitwise Operator/1 -> Conditionally Add State Info to Parm Info/1

== system CM340A_AdcDiagc/AdcDiagc/AdcDiagcPer1/Adc1 Diagc/State 0,2,4,6/State 4 ==
  Adc1SelfDiag0 : Inport  RequirementInfo={} %GIDa_f40f873b_8eb4_4df2_8933_d6a9347e94df
  Adc1SelfDiag2 : Inport  RequirementInfo={} %GIDa_5c394e8e_e398_4661_a357_19767f6ddc27  Port=2
  Adc1SelfDiag4 : Inport  RequirementInfo={} %GIDa_503a0d58_323d_421d_bbda_1621fa99bd96  Port=3
  DiagState : Inport  Port=4
  Action Port : ActionPort  ActionType=elseif
  Accuracy Check2 : CM340A_AdcDiagc_Library/Accuracy Check  RequirementInfo="{'linktype_rmi_doors' '000079f2 (/ESG Group/FDD Module Requirements/EA4 Specific/CM340A_AdcDiagc)' '#CM340A_163' 'true' 'REQ:  CM340A_163' '' } %GIDa_eb37628c_9c83_4f26_9023_edd5a925673e"
  Bitwise Operator : simulink/Logic and Bit Operations/Bitwise Operator  logicop=OR  UseBitMask=off  NumInputPorts=3  BitMask=bin2dec('11011001')  BitMaskRealWorld=Stored Integer
  Conditionally Add State Info to Parm Info : CM340A_AdcDiagc_Library/Conditionally Add State Info to Parm Info  RequirementInfo="{'linktype_rmi_doors' '000079f2 (/ESG Group/FDD Module Requirements/EA4 Specific/CM340A_AdcDiagc)' '#CM340A_164' 'true' 'REQ:  CM340A_164' '' } %GIDa_1f578c8b_78e7_43ca_bb67_b42afba011fd"
  Constant2 : Constant  Value=ADCDIAG4REFVOLT_VOLT_F32
  CopyRight2 : Subsystem  Description=|  mask(Copyright Information){none=on}
      | Copyright info block.                                               
      |                                                                     
      | Place copyright information at the top of every subsystem in design.
      mask prompts: none "No parameters"
      mask help: Place copyright information at the top of every subsystem in design.
      mask Display:
      | NxtrConf = 'Nexteer Confidential';
      | 
      | sys = bdroot; %handle for the current model ("system")
      | first = get_param(sys,'Created');
      | first = first(end-3:end);  %year is last four digits
      | 
      | last = get_param(sys,'LastModifiedDate');
      | if isempty(last)
      |     last = datestr(now,'yyyy');
      | else
      |     last = last(end-3:end);
      | end
      | 
      | if strcmp(first,last)
      |     fprintf('%s -- Copyright %s Nexteer',NxtrConf,first)
      | else
      |     fprintf('%s -- %s%s- %s Nexteer',NxtrConf,char(169),first,last)
      | end
  Data Store Read : DataStoreRead  DataStoreName=Adc1FltCntSt4
  Data Store Write : DataStoreWrite  DataStoreName=Adc1FltCntSt4
  Subsystem : Subsystem
  Zero Check : CM340A_AdcDiagc_Library/Zero Check  RequirementInfo="{'linktype_rmi_doors' '000079f2 (/ESG Group/FDD Module Requirements/EA4 Specific/CM340A_AdcDiagc)' '#CM340A_160' 'true' 'REQ:  CM340A_160' '' } %GIDa_71e3252b_e4ef_40f1_889a_82004b9cf866"
  Zero Check1 : CM340A_AdcDiagc_Library/Zero Check  RequirementInfo="{'linktype_rmi_doors' '000079f2 (/ESG Group/FDD Module Requirements/EA4 Specific/CM340A_AdcDiagc)' '#CM340A_162' 'true' 'REQ:  CM340A_162' '' } %GIDa_5e2e4837_71fd_4e5e_ab98_b6ce79d7bdad"
  Parameter Byte : Outport
  wires:
  DiagState/1 -> Conditionally Add State Info to Parm Info/2
  Bitwise Operator/1 -> Conditionally Add State Info to Parm Info/1
  Adc1SelfDiag0/1 -> Zero Check/1
  Adc1SelfDiag2/1 -> Zero Check1/1
  Adc1SelfDiag4/1 -> Accuracy Check2/1
  Constant2/1 -> Accuracy Check2/2
  Zero Check/1 -> Bitwise Operator/1
  Zero Check1/1 -> Bitwise Operator/2
  Accuracy Check2/1 -> Bitwise Operator/3
  Conditionally Add State Info to Parm Info/1 -> Subsystem/1(Parameter Byte), Parameter Byte/1
  Subsystem/1(FltCntr) -> Data Store Write/1
  Data Store Read/1 -> Subsystem/2(FltCntrPrev)

== system CM340A_AdcDiagc/AdcDiagc/AdcDiagcPer1/Adc1 Diagc/State 0,2,4,6/State 6 ==
  Adc1SelfDiag0 : Inport  RequirementInfo={} %GIDa_9e8b0eb5_33c3_4165_8f0d_938680b0487e
  Adc1SelfDiag2 : Inport  RequirementInfo={} %GIDa_54c08715_06ff_4351_84bc_27385d7ee22f  Port=2
  Adc1SelfDiag4 : Inport  RequirementInfo={} %GIDa_721d0ee1_e1aa_479d_8ab0_923ef2385a14  Port=3
  DiagState : Inport  Port=4
  Action Port : ActionPort  ActionType=else
  Accuracy Check1 : CM340A_AdcDiagc_Library/Accuracy Check  RequirementInfo="{'linktype_rmi_doors' '000079f2 (/ESG Group/FDD Module Requirements/EA4 Specific/CM340A_AdcDiagc)' '#CM340A_171' 'true' 'REQ:  CM340A_171' '' } %GIDa_52b97226_34cb_499c_b1b9_0699fa41f39a"
  Bitwise Operator : simulink/Logic and Bit Operations/Bitwise Operator  logicop=OR  UseBitMask=off  NumInputPorts=3  BitMask=bin2dec('11011001')  BitMaskRealWorld=Stored Integer
  Conditionally Add State Info to Parm Info : CM340A_AdcDiagc_Library/Conditionally Add State Info to Parm Info  RequirementInfo="{'linktype_rmi_doors' '000079f2 (/ESG Group/FDD Module Requirements/EA4 Specific/CM340A_AdcDiagc)' '#CM340A_173' 'true' 'REQ:  CM340A_173' '' } %GIDa_9fa6a2df_ef3b_402a_b9ef_4843e5fabdb5"
  Constant1 : Constant  Value=ADCDIAG2REFVOLT_VOLT_F32
  CopyRight2 : Subsystem  Description=|  mask(Copyright Information){none=on}
      | Copyright info block.                                               
      |                                                                     
      | Place copyright information at the top of every subsystem in design.
      mask prompts: none "No parameters"
      mask help: Place copyright information at the top of every subsystem in design.
      mask Display:
      | NxtrConf = 'Nexteer Confidential';
      | 
      | sys = bdroot; %handle for the current model ("system")
      | first = get_param(sys,'Created');
      | first = first(end-3:end);  %year is last four digits
      | 
      | last = get_param(sys,'LastModifiedDate');
      | if isempty(last)
      |     last = datestr(now,'yyyy');
      | else
      |     last = last(end-3:end);
      | end
      | 
      | if strcmp(first,last)
      |     fprintf('%s -- Copyright %s Nexteer',NxtrConf,first)
      | else
      |     fprintf('%s -- %s%s- %s Nexteer',NxtrConf,char(169),first,last)
      | end
  Data Store Read : DataStoreRead  DataStoreName=Adc1FltCntSt6
  Data Store Write : DataStoreWrite  DataStoreName=Adc1FltCntSt6
  Subsystem : Subsystem
  Zero Check : CM340A_AdcDiagc_Library/Zero Check  RequirementInfo="{'linktype_rmi_doors' '000079f2 (/ESG Group/FDD Module Requirements/EA4 Specific/CM340A_AdcDiagc)' '#CM340A_170' 'true' 'REQ:  CM340A_170' '' } %GIDa_c6b0cc90_f8c6_42c1_ab0d_7f3d6ea215ba"
  Zero Check1 : CM340A_AdcDiagc_Library/Zero Check  RequirementInfo="{'linktype_rmi_doors' '000079f2 (/ESG Group/FDD Module Requirements/EA4 Specific/CM340A_AdcDiagc)' '#CM340A_172' 'true' 'REQ:  CM340A_172' '' } %GIDa_b488c0f6_f5ea_4790_83e9_07684d3c49cf"
  Parameter Byte : Outport
  wires:
  Zero Check1/1 -> Bitwise Operator/3
  Accuracy Check1/1 -> Bitwise Operator/2
  Zero Check/1 -> Bitwise Operator/1
  Adc1SelfDiag4/1 -> Zero Check1/1
  Constant1/1 -> Accuracy Check1/2
  Adc1SelfDiag2/1 -> Accuracy Check1/1
  Adc1SelfDiag0/1 -> Zero Check/1
  Bitwise Operator/1 -> Conditionally Add State Info to Parm Info/1
  DiagState/1 -> Conditionally Add State Info to Parm Info/2
  Conditionally Add State Info to Parm Info/1 -> Subsystem/1(Parameter Byte), Parameter Byte/1
  Subsystem/1(FltCntr) -> Data Store Write/1
  Data Store Read/1 -> Subsystem/2(FltCntrPrev)

== system CM340A_AdcDiagc/AdcDiagc/AdcDiagcPer1/Adc1 Diagc/State 1,3,5,7/CopyRight2 ==

== system CM340A_AdcDiagc/AdcDiagc/AdcDiagcPer1/AdcDiagcPer2/Set Adc0ParFlt 0/CopyRight2 ==

== system CM340A_AdcDiagc/AdcDiagc/AdcDiagcPer1/AdcDiagcPer2/Set Adc0ParFlt to 0/CopyRight2 ==

== system CM340A_AdcDiagc/AdcDiagc/AdcDiagcPer1/AdcDiagcPer2/Set Adc0ParFlt to 128 and Err Clr Reg to 2/CopyRight2 ==

== system CM340A_AdcDiagc/AdcDiagc/AdcDiagcPer1/AdcDiagcPer2/Set Adc1ParFlt to 128 and Err Clr Reg to 4/CopyRight2 ==

== system CM340A_AdcDiagc/AdcDiagc/AdcDiagcPer1/NTC Fault Processing0/Atomic Subsystem/CopyRight2 ==

== system CM340A_AdcDiagc/AdcDiagc/AdcDiagcPer1/NTC Fault Processing0/Atomic Subsystem/Fail Step ==
  Action Port : ActionPort  ActionType=then
  Constant3 : Constant  Value=AdcDiagcNtc0x032FailStep
      settings: AttributesFormatString=Calibration
  CopyRight2 : Subsystem  Description=|  mask(Copyright Information){none=on}
      | Copyright info block.                                               
      |                                                                     
      | Place copyright information at the top of every subsystem in design.
      mask prompts: none "No parameters"
      mask help: Place copyright information at the top of every subsystem in design.
      mask Display:
      | NxtrConf = 'Nexteer Confidential';
      | 
      | sys = bdroot; %handle for the current model ("system")
      | first = get_param(sys,'Created');
      | first = first(end-3:end);  %year is last four digits
      | 
      | last = get_param(sys,'LastModifiedDate');
      | if isempty(last)
      |     last = datestr(now,'yyyy');
      | else
      |     last = last(end-3:end);
      | end
      | 
      | if strcmp(first,last)
      |     fprintf('%s -- Copyright %s Nexteer',NxtrConf,first)
      | else
      |     fprintf('%s -- %s%s- %s Nexteer',NxtrConf,char(169),first,last)
      | end
  NtcNr1 : simulink/Sources/Enumerated Constant  OutDataTypeStr=Enum: NtcSts1  Value=NtcSts1.NTCSTS_PREFAILD  SampleTime=inf
  NtcSts : Outport
  DebStep : Outport  Port=2
  wires:
  NtcNr1/1 -> NtcSts/1
  Constant3/1 -> DebStep/1

== system CM340A_AdcDiagc/AdcDiagc/AdcDiagcPer1/NTC Fault Processing0/Atomic Subsystem/Pass Step ==
  Action Port : ActionPort  ActionType=else
  Constant3 : Constant  Value=AdcDiagcNtc0x032PassStep
      settings: AttributesFormatString=Calibration
  CopyRight2 : Subsystem  Description=|  mask(Copyright Information){none=on}
      | Copyright info block.                                               
      |                                                                     
      | Place copyright information at the top of every subsystem in design.
      mask prompts: none "No parameters"
      mask help: Place copyright information at the top of every subsystem in design.
      mask Display:
      | NxtrConf = 'Nexteer Confidential';
      | 
      | sys = bdroot; %handle for the current model ("system")
      | first = get_param(sys,'Created');
      | first = first(end-3:end);  %year is last four digits
      | 
      | last = get_param(sys,'LastModifiedDate');
      | if isempty(last)
      |     last = datestr(now,'yyyy');
      | else
      |     last = last(end-3:end);
      | end
      | 
      | if strcmp(first,last)
      |     fprintf('%s -- Copyright %s Nexteer',NxtrConf,first)
      | else
      |     fprintf('%s -- %s%s- %s Nexteer',NxtrConf,char(169),first,last)
      | end
  NtcNr1 : simulink/Sources/Enumerated Constant  OutDataTypeStr=Enum: NtcSts1  Value=NtcSts1.NTCSTS_PREPASSD  SampleTime=inf
  NtcSts : Outport
  DebStep : Outport  Port=2
  wires:
  Constant3/1 -> DebStep/1
  NtcNr1/1 -> NtcSts/1

== system CM340A_AdcDiagc/AdcDiagc/AdcDiagcPer1/NTC Fault Processing0/GetNtcQlfr/CopyRight2 ==

== system CM340A_AdcDiagc/AdcDiagc/AdcDiagcPer1/NTC Fault Processing0/SetNtcSts/CopyRight2 ==

== system CM340A_AdcDiagc/AdcDiagc/AdcDiagcPer1/NTC Fault Processing0/SetNtcSts/Enabled Subsystem ==
  In1 : Inport
  Enable : EnablePort
  Bitwise Operator : simulink/Logic and Bit Operations/Bitwise Operator  logicop=OR  UseBitMask=off  NumInputPorts=2  BitMask=bin2dec('11011001')  BitMaskRealWorld=Stored Integer
  CopyRight2 : Subsystem  Description=|  mask(Copyright Information){none=on}
      | Copyright info block.                                               
      |                                                                     
      | Place copyright information at the top of every subsystem in design.
      mask prompts: none "No parameters"
      mask help: Place copyright information at the top of every subsystem in design.
      mask Display:
      | NxtrConf = 'Nexteer Confidential';
      | 
      | sys = bdroot; %handle for the current model ("system")
      | first = get_param(sys,'Created');
      | first = first(end-3:end);  %year is last four digits
      | 
      | last = get_param(sys,'LastModifiedDate');
      | if isempty(last)
      |     last = datestr(now,'yyyy');
      | else
      |     last = last(end-3:end);
      | end
      | 
      | if strcmp(first,last)
      |     fprintf('%s -- Copyright %s Nexteer',NxtrConf,first)
      | else
      |     fprintf('%s -- %s%s- %s Nexteer',NxtrConf,char(169),first,last)
      | end
  Data Store Read : DataStoreRead  DataStoreName=Adc0DynDiagcPrm
  Data Store Write1 : DataStoreWrite  DataStoreName=Adc0DynDiagcPrm
  wires:
  In1/1 -> Bitwise Operator/1
  Bitwise Operator/1 -> Data Store Write1/1
  Data Store Read/1 -> Bitwise Operator/2

== system CM340A_AdcDiagc/AdcDiagc/AdcDiagcPer1/NTC Fault Processing1/Atomic Subsystem/CopyRight2 ==
